simulink model "lap2part3"  (R2021a)
settings: Solver=VariableStepAuto  StartTime=0.0  StopTime=10.0  RelTol=1e-3
libraries: dsparch4 x1
settings Model: Creator=USER59  LastModifiedBy=USER59

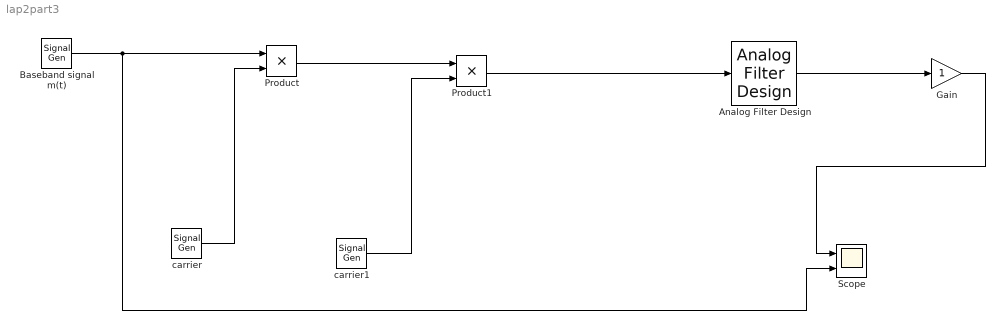
== system lap2part3 ==
  Analog Filter Design : dsparch4/Analog Filter Design  method=Butterworth  filttype=Lowpass  N=8  Wlo=30  Whi=80  Rp=2  Rs=40
  Baseband signal m(t) : SignalGenerator  Frequency=4000  Units=rad/sec
  Gain : Gain
  Product : Product
  Product1 : Product
  Scope : Scope  NumInputPorts=2
  carrier : SignalGenerator  Frequency=20000  Units=rad/sec
  carrier1 : SignalGenerator  Frequency=20000  Units=rad/sec
  wires:
  carrier/1 -> Product/2
  Baseband signal m(t)/1 -> Scope/2, Product/1
  Product/1 -> Product1/1
  carrier1/1 -> Product1/2
  Product1/1 -> Analog Filter Design/1
  Analog Filter Design/1 -> Gain/1
  Gain/1 -> Scope/1
